simulink model "transfer_f"  (R2023b)
settings: Solver=FixedStepAuto  StartTime=0.0  StopTime=10.0  FixedStep=0.0005  RelTol=1e-3
values from neighbouring files (symbols this model uses):
  B = 0.0003    [transfer.m]
  H = (N1(1)-D1(3))/N1(1)    [transfer.m]
  J = 2.09*10^(-5)    (= 2.09e-05)    [transfer.m]
  Kb = 0.042    [transfer.m]
  Kt = 0.042    [transfer.m]
  L = 1.16    [transfer.m]
  R = 8.4    [transfer.m]
settings Model: Creator=yeoseojeong  LastModifiedBy=yeoseojeong

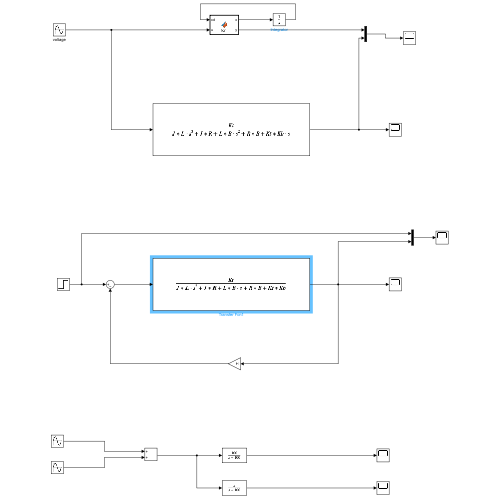
[thumbnail: Simulink's stored preview of the top-level diagram]
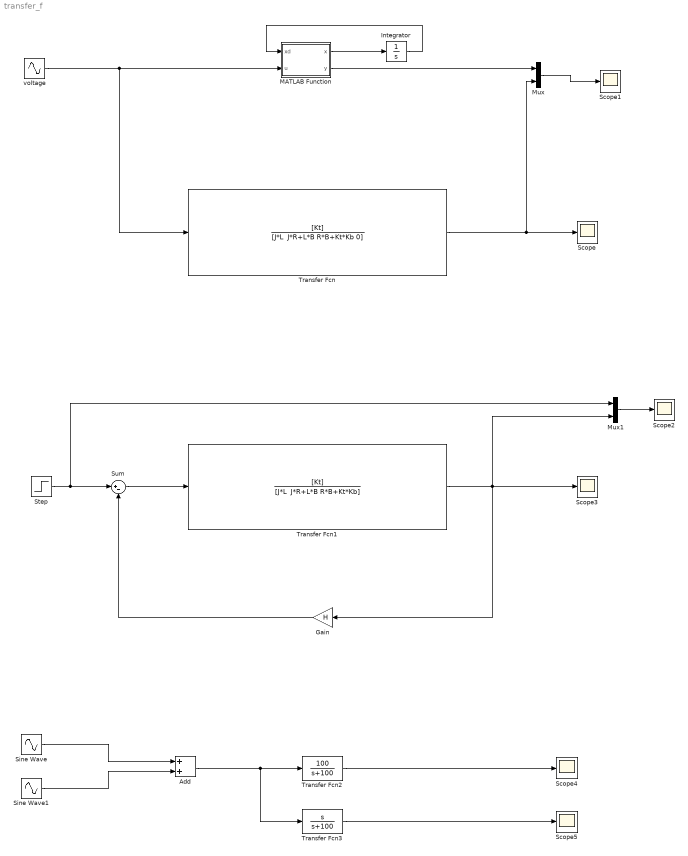
== system transfer_f ==
  Add : Sum
  Gain : Gain  Gain=H
  Integrator : Integrator
  MATLAB Function : MATLAB Function  TreatAsAtomicUnit=on
  Mux : Mux  Inputs=2
  Mux1 : Mux  Inputs=2
  Scope{,1..5} (6 alike) : Scope
  Sine Wave : Sin  SampleTime=0
  Sine Wave1 : Sin  Frequency=1000  SampleTime=0
  Step : Step  SampleTime=0
  Sum : Sum  Inputs=|+-
  Transfer Fcn : TransferFcn  Numerator=[Kt]  Denominator="[J*L  J*R+L*B R*B+Kt*Kb 0]"
  Transfer Fcn1 : TransferFcn  Numerator=[Kt]  Denominator="[J*L  J*R+L*B R*B+Kt*Kb]"
  Transfer Fcn2 : TransferFcn  Numerator=[100]  Denominator=[1 100]
  Transfer Fcn3 : TransferFcn  Numerator=[1 0]  Denominator=[1 100]
  voltage : Sin  SampleTime=0
  wires:
  Integrator/1 -> MATLAB Function/1(xd)
  MATLAB Function/1(x) -> Integrator/1
  Mux/1 -> Scope1/1
  Transfer Fcn/1 -> Mux/2, Scope/1
  voltage/1 -> MATLAB Function/2(u), Transfer Fcn/1
  MATLAB Function/2(y) -> Mux/1
  Step/1 -> Mux1/1, Sum/1
  Sum/1 -> Transfer Fcn1/1
  Gain/1 -> Sum/2
  Mux1/1 -> Scope2/1
  Transfer Fcn1/1 -> Gain/1, Mux1/2, Scope3/1
  Add/1 -> Transfer Fcn3/1, Transfer Fcn2/1
  Sine Wave/1 -> Add/1
  Sine Wave1/1 -> Add/2
  Transfer Fcn3/1 -> Scope5/1
  Transfer Fcn2/1 -> Scope4/1

== matlab function transfer_f/MATLAB Function ==
  data: xd input size=3; x output; y output; u input
function [x,y] = fcn(xd,u)

J=2.09*10^(-5); %kg m 2
Kb=0.042;
Kt=0.042;
R=8.4;
L=1.16;
B=0.0003;


x=[xd(2);
    Kt/J*xd(3)-B/J*xd(2);
    -R/L*xd(3)-Kb/L*xd(2)+1/L*u];

y=xd(1);
